simulink model "BPSK_b"  (Simulink 6.3)
settings: Solver=ode45  StartTime=0.0  StopTime=100  RelTol=1e-3
libraries: xbsIndex_r4 x7, commrandsrc2 x1
settings Model: LastModifiedBy=Administrador

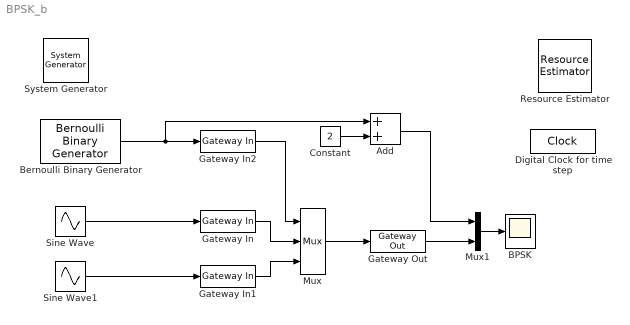
== system BPSK_b ==
  " System Generator" : xbsIndex_r4/ System Generator  Tag=genX  xilinxfamily=Virtex4  part=xc4vsx35  speed=-10  package=ff668  synthesis_tool=XST  directory=./netlist  testbench=off  simulink_period=1/20  sysclk_period=10  incr_netlist=off  trim_vbits=Everywhere in SubSystem  dbl_ovrd=According to Block Masks  core_generation=According to Block Masks  run_coregen=off  deprecated_control=off  eval_field=0  block_type=sysgen
  Add : Sum  OutScaling=2^-10
  BPSK : Scope
      settings: YMin=-2  YMax=4
  Bernoulli Binary Generator : commrandsrc2/Bernoulli Binary Generator  P=0.5  seed=61  Ts=5  frameBased=off  sampPerFrame=1  orient=off  outDataType=double
  Constant : Constant  Value=2
  Digital Clock for time step : DigitalClock  SampleTime=0.00005
  Gateway In : xbsIndex_r4/Gateway In  arith_type="Signed  (2's comp)"  n_bits=6  bin_pt=4  quantization="Round  (unbiased: +/- Inf)"  overflow=Saturate  period=1/20  dbl_ovrd=off  timing_constraint=None  locs_specified=off  LOCs={}  block_type=gatewayin
      settings: infoedit="Gateway in block.  Converts inputs of type Simulink integer, double and fixed point to  Xilinx fixed point type.<P><P>Hardware notes:  In hardware these blocks become top level input ports."  block_version=VER_STRING_GOES_HERE
  Gateway In1 : xbsIndex_r4/Gateway In  arith_type="Signed  (2's comp)"  n_bits=6  bin_pt=4  quantization="Round  (unbiased: +/- Inf)"  overflow=Saturate  period=1/20  dbl_ovrd=off  timing_constraint=None  locs_specified=off  LOCs={}  block_type=gatewayin
      settings: infoedit="Gateway in block.  Converts inputs of type Simulink integer, double and fixed point to  Xilinx fixed point type.<P><P>Hardware notes:  In hardware these blocks become top level input ports."  block_version=VER_STRING_GOES_HERE
  Gateway In2 : xbsIndex_r4/Gateway In  arith_type=Boolean  n_bits=16  bin_pt=14  quantization="Round  (unbiased: +/- Inf)"  overflow=Saturate  period=1  dbl_ovrd=off  timing_constraint=None  locs_specified=off  LOCs={}  block_type=gatewayin
      settings: infoedit="Gateway in block.  Converts inputs of type Simulink integer, double and fixed point to  Xilinx fixed point type.<P><P>Hardware notes:  In hardware these blocks become top level input ports."  block_version=VER_STRING_GOES_HERE
  Gateway Out : xbsIndex_r4/Gateway Out  hdl_port=on  timing_constraint=None  locs_specified=off  LOCs={}  block_type=gatewayout
      settings: infoedit="Gateway out block.  Converts Xilinx fixed point inputs into ouputs of type Simulink integer, double, or fixed point.<P><P>Hardware notes:  In hardware these blocks become top level output ports or are discarded, depending on how they are configured."  block_version=VER_STRING_GOES_HERE
  Mux : xbsIndex_r4/Mux  inputs=2  en=off  latency=0  precision=Full  arith_type=Unsigned  n_bits=16  bin_pt=14  quantization=Truncate  overflow=Wrap  dbl_ovrd=off  block_type=mux
      settings: block_version=VER_STRING_GOES_HERE
  Mux1 : Mux  Inputs=2
  Resource Estimator : xbsIndex_r4/Resource Estimator  Tag=resEstTag  Slices=0  FFs=0  BRAMs=0  LUTs=0  IOBs=0  EBMs=0  TBUFs=0  xl_use_estimator_area=off  est_options=Estimate  block_type=resource_estimator
      settings: AttributesFormatString=Resource\nEstimator
  Sine Wave : Sin  SineType=Sample based  Samples=100  SampleTime=1/20
  Sine Wave1 : Sin  SineType=Sample based  Samples=100  SampleTime=1/20  Offset=50
  wires:
  Sine Wave/1 -> Gateway In/1
  Sine Wave1/1 -> Gateway In1/1
  Gateway In/1 -> Mux/2
  Gateway In1/1 -> Mux/3
  Mux/1 -> Gateway Out/1
  Gateway In2/1 -> Mux/1
  Bernoulli Binary Generator/1 -> Gateway In2/1, Add/1
  Constant/1 -> Add/2
  Gateway Out/1 -> Mux1/2
  Add/1 -> Mux1/1
  Mux1/1 -> BPSK/1
